simulink library "Lib_PF_BusGenAC_TMATS"  (R2017a)
settings: Solver=ode45  StartTime=0.0  StopTime=10.0  RelTol=1e-3  EnableMultiTasking=on
Description:
  | Thomas Modules
settings Model: Creator=jwchapm2  LastModifiedBy=glthoma1
settings DataIOCC: LimitDataPoints=on  SaveFormat=Array
settings OptimizationCC: ExpressionDepthLimit=2147483647  LifeSpan=inf
settings DebuggingCC: UnderspecifiedInitializationDetection=Classic  MergeDetectMultiDrivingBlocksExec=none  SolverPrmCheckMsg=warning  StateNameClashWarn=warning  SFUnexpectedBacktrackingDiag=warning  SFNoUnconditionalDefaultTransitionDiag=warning  SFExecutionAtInitializationDiag=none
settings HardwareCC: ProdBitPerPointer=32  ProdBitPerSizeT=32  ProdBitPerPtrDiffT=32  ProdLargestAtomicFloat=None  ProdIntDivRoundTo=Undefined  ProdEndianess=Unspecified  ProdWordSize=32  ProdHWDeviceType=32-bit Generic
settings ModelReferenceCC: PropagateSignalLabelsOutOfModel=off
settings GRTTargetCC: TargetLangStandard=C89/C90 (ANSI)  GeneratePreprocessorConditionals=Disable all
settings ConfigComp: CovMetricSettings=dw  CovHtmlReporting=on  CovSaveCumulativeToWorkspaceVar=on  CovSaveSingleToWorkspaceVar=on  CovExternalEMLEnable=off

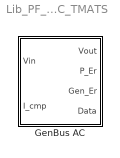
== system Lib_PF_BusGenAC_TMATS ==
  GenBus AC : Subsystem  mask{PeInEN_M=off, BlkNm_M=double(gcb), Vispec_M=1.04, P_M=2, Qmax_M=100, Qmin_M=-100}
      mask prompts: PeInEN_M "PelInEN_M - External Pelec"; BlkNm_M "Block name as double"; Vispec_M "Vispec_M - specified absolute vlaue of voltage"; P_M "P_M - generated real power"; Qmax_M "Qmax_M - max reactive power"; Qmin_M "Qmin_M - min reactive power"
      mask init:
      | %Manage Power Inputs
      | if PeInEN_M == 1
      |     if strcmp(get_param([BlkNm_M '/Pelec'],'BlockType'),'Constant')
      |         MSK_ReplaceBlock_TMATS([BlkNm_M '/Pelec'],'built-in/Inport');
      |     end
      |     set_param([BlkNm_M '/Pelec'],'Port',num2str(2));
      | elseif PeInEN_M == 0
      |     if strcmp(get_param([BlkNm_M '/Pelec'],'BlockType'),'Inport')
      |         MSK_ReplaceBlock_TMATS([BlkNm_M '/Pelec'],'built-in/Constant');
      |         set_param([BlkNm_M '/Pelec'],'Value','P_M');
      |     end
      | end
      mask Callback PeInEN_M: MSK_SEC_Enables_TMATS('PeInEN_M',4,'dis')

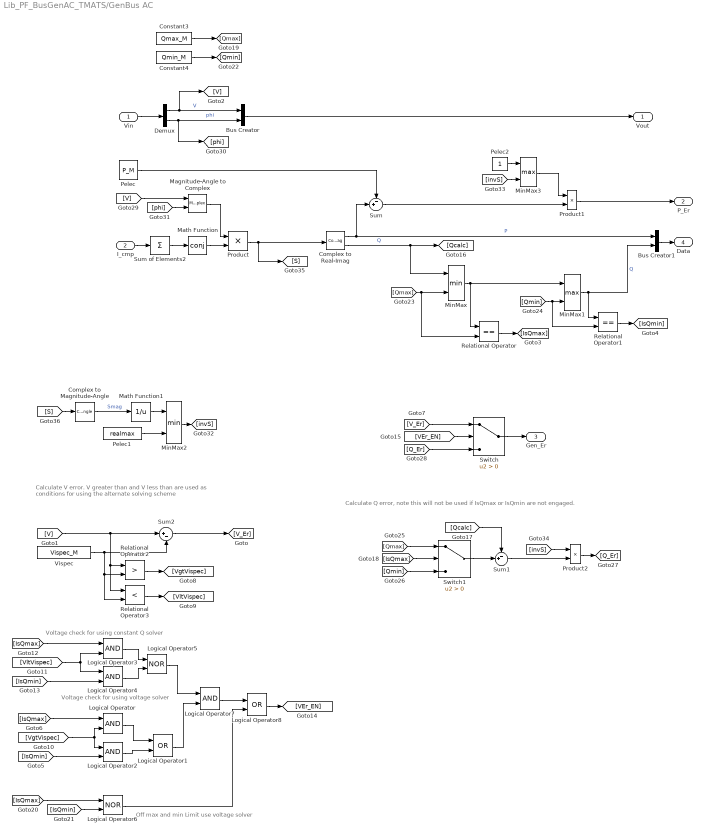
== system Lib_PF_BusGenAC_TMATS/GenBus AC ==
  note: Calculate V error.  V greater than and V less than are used as
      | conditions for using the alternate solving scheme
  note: Voltage check for using constant Q solver
  note: Voltage check for using voltage solver
  note: Off max and min Limit use voltage solver
  note: Calculate Q error, note this will not be used if IsQmax or IsQmin are not engaged.
  Vin : Inport
  I_cmp : Inport  Port=2
  Bus Creator : BusCreator  Inputs=2
  Bus Creator1 : BusCreator  Inputs=2
  Complex to Magnitude-Angle : ComplexToMagnitudeAngle  Output=Magnitude
  Complex to Real-Imag : ComplexToRealImag
  Constant3 : Constant  Value=Qmax_M
  Constant4 : Constant  Value=Qmin_M
  Demux : Demux  Outputs=2
  Logical Operator{,2..4,7} (5 alike) : Logic  AllPortsSameDT=off  OutDataTypeStr=boolean
  Logical Operator1 : Logic  Operator=OR  AllPortsSameDT=off  OutDataTypeStr=boolean
  Logical Operator5 : Logic  Operator=NOR  AllPortsSameDT=off  OutDataTypeStr=boolean
  Logical Operator6 : Logic  Operator=NOR  AllPortsSameDT=off  OutDataTypeStr=boolean
  Logical Operator8 : Logic  Operator=OR  AllPortsSameDT=off  OutDataTypeStr=boolean
  Magnitude-Angle to Complex : MagnitudeAngleToComplex
  Math Function : Math  Operator=conj  SaturateOnIntegerOverflow=on
  Math Function1 : Math  Operator=reciprocal  SaturateOnIntegerOverflow=on
  MinMax : MinMax  Inputs=2
  MinMax1 : MinMax  Function=max  Inputs=2
  MinMax2 : MinMax  Inputs=2
  MinMax3 : MinMax  Function=max  Inputs=2
  Pelec : Constant  Value=P_M
  Pelec1 : Constant  Value=realmax
  Pelec2 : Constant
  Product : Product
  Product1 : Product
  Product2 : Product
  Relational Operator : RelationalOperator  Operator===  OutDataTypeStr=boolean  RndMeth=Nearest
  Relational Operator1 : RelationalOperator  Operator===  OutDataTypeStr=boolean  RndMeth=Nearest
  Relational Operator2 : RelationalOperator  Operator=>  OutDataTypeStr=boolean  RndMeth=Nearest
  Relational Operator3 : RelationalOperator  Operator=<  OutDataTypeStr=boolean  RndMeth=Nearest
  Sum : Sum  Inputs=-+|
  Sum of Elements2 : Sum  Inputs=+
  Sum1 : Sum  Inputs=-+|
  Sum2 : Sum  Inputs=|+-
  Switch : Switch  Criteria=u2 > Threshold
  Switch1 : Switch  Criteria=u2 > Threshold
  Vispec : Constant  Value=Vispec_M
  Vout : Outport
  P_Er : Outport  Port=2
  Gen_Er : Outport  Port=3
  Data : Outport  Port=4
  wires:
  Logical Operator7/1 -> Logical Operator8/1
  [phi] -> Magnitude-Angle to Complex/2
  [V] -> Magnitude-Angle to Complex/1
  [Q_Er] -> Switch/3
  Sum1/1 -> Product2/2
  [Qcalc] -> Sum1/1
  Switch1/1 -> Sum1/2
  [Qmin] -> Switch1/3
  [Qmax] -> Switch1/1
  Constant4/1 -> [Qmin]
  Constant3/1 -> [Qmax]
  [Qmin] -> MinMax1/2, Relational Operator1/2
  [Qmax] -> MinMax/2, Relational Operator/2
  [IsQmax] -> Switch1/2
  Logical Operator6/1 -> Logical Operator8/2
  [IsQmin] -> Logical Operator6/2
  [IsQmax] -> Logical Operator6/1
  [VEr_EN] -> Switch/2
  Logical Operator8/1 -> [VEr_EN]
  Logical Operator5/1 -> Logical Operator7/1
  Logical Operator1/1 -> Logical Operator7/2
  Switch/1 -> Gen_Er/1
  [V_Er] -> Switch/1
  Logical Operator2/1 -> Logical Operator1/2
  Logical Operator/1 -> Logical Operator1/1
  Logical Operator4/1 -> Logical Operator5/2
  Logical Operator3/1 -> Logical Operator5/1
  [IsQmin] -> Logical Operator4/2
  [IsQmax] -> Logical Operator3/1
  [IsQmin] -> Logical Operator2/2
  [VltVispec] -> Logical Operator4/1, Logical Operator3/2
  [IsQmax] -> Logical Operator/1
  [VgtVispec] -> Logical Operator/2, Logical Operator2/1
  Relational Operator2/1 -> [VgtVispec]
  Relational Operator3/1 -> [VltVispec]
  Relational Operator1/1 -> [IsQmin]
  Relational Operator/1 -> [IsQmax]
  MinMax1/1 -> Relational Operator1/1, Bus Creator1/2  "Q"
  MinMax/1 -> Relational Operator/1, MinMax1/1
  Math Function/1 -> Product/2
  Magnitude-Angle to Complex/1 -> Product/1
  Sum of Elements2/1 -> Math Function/1
  I_cmp/1 -> Sum of Elements2/1
  Complex to Real-Imag/2 -> MinMax/1, [Qcalc]  "Q"
  Complex to Real-Imag/1 -> Bus Creator1/1, Sum/2  "P"
  Demux/2 -> Bus Creator/2, [phi]  "phi"
  Demux/1 -> Bus Creator/1, [V]  "V"
  Vin/1 -> Demux/1
  Vispec/1 -> Sum2/2, Relational Operator2/2, Relational Operator3/2
  Bus Creator/1 -> Vout/1
  Pelec/1 -> Sum/1
  Bus Creator1/1 -> Data/1
  Product/1 -> [S], Complex to Real-Imag/1
  Complex to Magnitude-Angle/1 -> Math Function1/1  "Smag"
  Math Function1/1 -> MinMax2/1
  Sum/1 -> Product1/2
  [invS] -> Product2/1
  Product2/1 -> [Q_Er]
  [V] -> Relational Operator2/1, Relational Operator3/1, Sum2/1
  Sum2/1 -> [V_Er]
  MinMax2/1 -> [invS]
  Pelec1/1 -> MinMax2/2
  [S] -> Complex to Magnitude-Angle/1
  [invS] -> MinMax3/2
  MinMax3/1 -> Product1/1
  Pelec2/1 -> MinMax3/1
  Product1/1 -> P_Er/1
